simulink model "AariaHIABTorqueR2017a2"  (R2017a)
settings: Solver=VariableStepAuto  StartTime=0.0  StopTime=inf  FixedStep=0.1  RelTol=1e-3  EnableMultiTasking=on
model workspace (MATLAB code in the model file):
  | my_a =1;
undefined symbols (not defined in the file or in its folder): AARIAENV, AARIAMAN, AARIASEN, Camera, sensor, Source_TS, X, Y, Z
libraries: sm_lib x369, nesl_utility x225, dspmathops x92, simulink x70, powerlib_meascontrol x3, vrlib x2, aerolibanimutils x1, aerolibutil x1
(part 6 of 10)

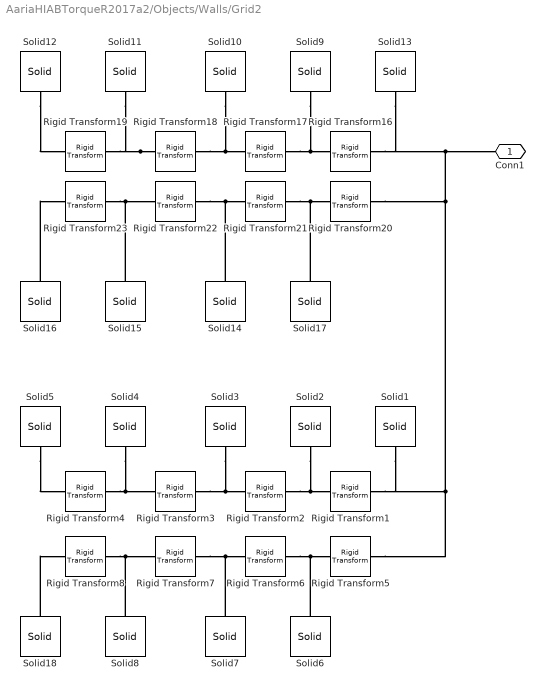
== system AariaHIABTorqueR2017a2/Objects/Walls/Grid2 ==
  Rigid Transform{1..4} (4 alike) : sm_lib/Frames and Transforms/Rigid Transform  TranslationMethod=StandardAxis  TranslationStandardOffset=2  TranslationLengthUnit=m  TranslationStandardAxis=+Y  TranslationCartesianOffset=[0 0 0]  TranslationROffset=0  TranslationROffsetUnits=m  TranslationZOffset=0  TranslationZOffsetUnits=m  TranslationThetaOffset=0  TranslationThetaOffsetUnits=deg  RotationMethod=None  RotationAngleUnits=deg  RotationStandardAxis=+Z  RotationAngle=0.0  RotationArbitraryAxis=[0 0 1]  FollAlignAxisA=+X  BaseAlignAxisA=+Y  FollAlignAxisB=+Y  BaseAlignAxisB=+Z  RotationSequenceAxes=FollowerAxes  RotationSequence=XYX  RotationSequenceAngles=[0 0 0]  RotationSequenceAnglesUnits=deg  RotationMatrix=[1 0 0; 0 1 0; 0 0 1]
  Rigid Transform{16..19} (4 alike) : sm_lib/Frames and Transforms/Rigid Transform  TranslationMethod=StandardAxis  TranslationStandardOffset=2  TranslationLengthUnit=m  TranslationStandardAxis=+X  TranslationCartesianOffset=[0 0 0]  TranslationROffset=0  TranslationROffsetUnits=m  TranslationZOffset=0  TranslationZOffsetUnits=m  TranslationThetaOffset=0  TranslationThetaOffsetUnits=deg  RotationMethod=None  RotationAngleUnits=deg  RotationStandardAxis=+Z  RotationAngle=0.0  RotationArbitraryAxis=[0 0 1]  FollAlignAxisA=+X  BaseAlignAxisA=+Y  FollAlignAxisB=+Y  BaseAlignAxisB=+Z  RotationSequenceAxes=FollowerAxes  RotationSequence=XYX  RotationSequenceAngles=[0 0 0]  RotationSequenceAnglesUnits=deg  RotationMatrix=[1 0 0; 0 1 0; 0 0 1]
  Rigid Transform{20..23} (4 alike) : sm_lib/Frames and Transforms/Rigid Transform  TranslationMethod=StandardAxis  TranslationStandardOffset=2  TranslationLengthUnit=m  TranslationStandardAxis=-X  TranslationCartesianOffset=[0 0 0]  TranslationROffset=0  TranslationROffsetUnits=m  TranslationZOffset=0  TranslationZOffsetUnits=m  TranslationThetaOffset=0  TranslationThetaOffsetUnits=deg  RotationMethod=None  RotationAngleUnits=deg  RotationStandardAxis=+Z  RotationAngle=0.0  RotationArbitraryAxis=[0 0 1]  FollAlignAxisA=+X  BaseAlignAxisA=+Y  FollAlignAxisB=+Y  BaseAlignAxisB=+Z  RotationSequenceAxes=FollowerAxes  RotationSequence=XYX  RotationSequenceAngles=[0 0 0]  RotationSequenceAnglesUnits=deg  RotationMatrix=[1 0 0; 0 1 0; 0 0 1]
  Rigid Transform{5..8} (4 alike) : sm_lib/Frames and Transforms/Rigid Transform  TranslationMethod=StandardAxis  TranslationStandardOffset=2  TranslationLengthUnit=m  TranslationStandardAxis=-Y  TranslationCartesianOffset=[0 0 0]  TranslationROffset=0  TranslationROffsetUnits=m  TranslationZOffset=0  TranslationZOffsetUnits=m  TranslationThetaOffset=0  TranslationThetaOffsetUnits=deg  RotationMethod=None  RotationAngleUnits=deg  RotationStandardAxis=+Z  RotationAngle=0.0  RotationArbitraryAxis=[0 0 1]  FollAlignAxisA=+X  BaseAlignAxisA=+Y  FollAlignAxisB=+Y  BaseAlignAxisB=+Z  RotationSequenceAxes=FollowerAxes  RotationSequence=XYX  RotationSequenceAngles=[0 0 0]  RotationSequenceAnglesUnits=deg  RotationMatrix=[1 0 0; 0 1 0; 0 0 1]
  Solid{1..8,18} (9 alike) : sm_lib/Body Elements/Solid  InertiaType=CalculateFromGeometry  Mass=1  MassUnits=kg  CenterOfMass=[0 0 0]  CenterOfMassUnits=m  MomentsOfInertia=[1 1 1]  MomentsOfInertiaUnits=kg*m^2  ProductsOfInertia=[1 1 1]  ProductsOfInertiaUnits=kg*m^2  DensityBased=on  Density=1000  DensityUnits=kg/m^3  DoExposeReferenceFrame=on  SerializedFrames=<Frames/>  GraphicType=FromGeometry  MarkerShape=Sphere  MarkerSize=10  GraphicVisPropType=SimpleVisualProperties  GraphicDiffuseColor=[0.4 0.4 0.4]  GraphicSpecularColor=[0.5 0.5 0.5 1.0]  GraphicAmbientColor=[0.15 0.15 0.15 1.0]  GraphicEmissiveColor=[0.0 0.0 0.0 1.0]  GraphicShininess=75  GraphicOpacity=1.0  GeometryShape=Brick  RectangleSize=[1 1]  RectangleSizeUnits=m  BrickDimensions=[20 1 0.12]  BrickDimensionUnits=m  CylinderRadius=1  CylinderRadiusUnits=m  CylinderLength=1  CylinderLengthUnits=m  SphereRadius=1  SphereRadiusUnits=m  EllipsoidRadii=[1 1 1]  EllipsoidRadiiUnits=m  ExtrusionCrossSection=[1 1; -1 1; -1 -1; 1 -1]  ExtrusionCrossSectionUnits=m  ExtrusionLength=1  ExtrusionLengthUnits=m  PolygonNumSides=3  PolygonOuterRadius=1  PolygonOuterRadiusUnits=m  ExtGeomFileType=STEP  ExtGeomFileUnits=m  RevolutionCrossSection=[1 1; 1 -1; 2 -1; 2 1]  RevolutionCrossSectionUnits=m  RevolutionExtent=Full  RevolutionAngle=180  RevolutionAngleUnits=deg
  Solid{9..17} (9 alike) : sm_lib/Body Elements/Solid  InertiaType=CalculateFromGeometry  Mass=1  MassUnits=kg  CenterOfMass=[0 0 0]  CenterOfMassUnits=m  MomentsOfInertia=[1 1 1]  MomentsOfInertiaUnits=kg*m^2  ProductsOfInertia=[1 1 1]  ProductsOfInertiaUnits=kg*m^2  DensityBased=on  Density=1000  DensityUnits=kg/m^3  DoExposeReferenceFrame=on  SerializedFrames=<Frames/>  GraphicType=FromGeometry  MarkerShape=Sphere  MarkerSize=10  GraphicVisPropType=SimpleVisualProperties  GraphicDiffuseColor=[0.2 0.2 0.2]  GraphicSpecularColor=[0.5 0.5 0.5 1.0]  GraphicAmbientColor=[0.15 0.15 0.15 1.0]  GraphicEmissiveColor=[0.0 0.0 0.0 1.0]  GraphicShininess=75  GraphicOpacity=1.0  GeometryShape=Brick  RectangleSize=[1 1]  RectangleSizeUnits=m  BrickDimensions=[1 20 0.11]  BrickDimensionUnits=m  CylinderRadius=1  CylinderRadiusUnits=m  CylinderLength=1  CylinderLengthUnits=m  SphereRadius=1  SphereRadiusUnits=m  EllipsoidRadii=[1 1 1]  EllipsoidRadiiUnits=m  ExtrusionCrossSection=[1 1; -1 1; -1 -1; 1 -1]  ExtrusionCrossSectionUnits=m  ExtrusionLength=1  ExtrusionLengthUnits=m  PolygonNumSides=3  PolygonOuterRadius=1  PolygonOuterRadiusUnits=m  ExtGeomFileType=STEP  ExtGeomFileUnits=m  RevolutionCrossSection=[1 1; 1 -1; 2 -1; 2 1]  RevolutionCrossSectionUnits=m  RevolutionExtent=Full  RevolutionAngle=180  RevolutionAngleUnits=deg
  Conn1 : PMIOPort  Port=1  Side=Right
  connections:
  Solid12/RConn1 -- Rigid Transform19/RConn1
  Rigid Transform18/RConn1 -- Rigid Transform19/LConn1 -- Solid11/RConn1
  Rigid Transform5/LConn1 -- Rigid Transform20/LConn1 -- Conn1/RConn1 -- Solid13/RConn1 -- Rigid Transform16/LConn1 -- Rigid Transform1/LConn1 -- Solid1/RConn1
  Rigid Transform21/LConn1 -- Rigid Transform20/RConn1 -- Solid17/RConn1
  Rigid Transform18/LConn1 -- Rigid Transform17/RConn1 -- Solid10/RConn1
  Solid15/RConn1 -- Rigid Transform23/LConn1 -- Rigid Transform22/RConn1
  Rigid Transform22/LConn1 -- Solid14/RConn1 -- Rigid Transform21/RConn1
  Rigid Transform17/LConn1 -- Rigid Transform16/RConn1 -- Solid9/RConn1
  Solid16/RConn1 -- Rigid Transform23/RConn1
  Rigid Transform2/LConn1 -- Solid2/RConn1 -- Rigid Transform1/RConn1
  Rigid Transform3/LConn1 -- Solid3/RConn1 -- Rigid Transform2/RConn1
  Solid4/RConn1 -- Rigid Transform4/LConn1 -- Rigid Transform3/RConn1
  Solid5/RConn1 -- Rigid Transform4/RConn1
  Rigid Transform6/LConn1 -- Rigid Transform5/RConn1 -- Solid6/RConn1
  Rigid Transform7/LConn1 -- Solid7/RConn1 -- Rigid Transform6/RConn1
  Rigid Transform8/LConn1 -- Solid8/RConn1 -- Rigid Transform7/RConn1
  Solid18/RConn1 -- Rigid Transform8/RConn1

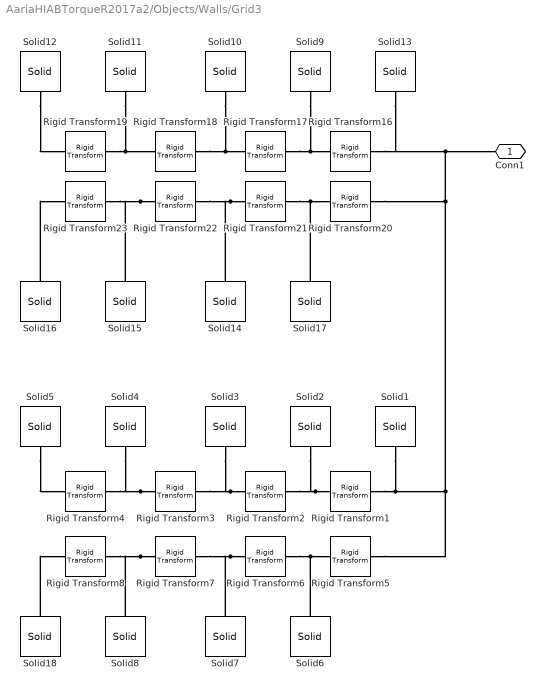
== system AariaHIABTorqueR2017a2/Objects/Walls/Grid3 ==
  Rigid Transform{1..4} (4 alike) : sm_lib/Frames and Transforms/Rigid Transform  TranslationMethod=StandardAxis  TranslationStandardOffset=2  TranslationLengthUnit=m  TranslationStandardAxis=+Y  TranslationCartesianOffset=[0 0 0]  TranslationROffset=0  TranslationROffsetUnits=m  TranslationZOffset=0  TranslationZOffsetUnits=m  TranslationThetaOffset=0  TranslationThetaOffsetUnits=deg  RotationMethod=None  RotationAngleUnits=deg  RotationStandardAxis=+Z  RotationAngle=0.0  RotationArbitraryAxis=[0 0 1]  FollAlignAxisA=+X  BaseAlignAxisA=+Y  FollAlignAxisB=+Y  BaseAlignAxisB=+Z  RotationSequenceAxes=FollowerAxes  RotationSequence=XYX  RotationSequenceAngles=[0 0 0]  RotationSequenceAnglesUnits=deg  RotationMatrix=[1 0 0; 0 1 0; 0 0 1]
  Rigid Transform{16..19} (4 alike) : sm_lib/Frames and Transforms/Rigid Transform  TranslationMethod=StandardAxis  TranslationStandardOffset=2  TranslationLengthUnit=m  TranslationStandardAxis=+X  TranslationCartesianOffset=[0 0 0]  TranslationROffset=0  TranslationROffsetUnits=m  TranslationZOffset=0  TranslationZOffsetUnits=m  TranslationThetaOffset=0  TranslationThetaOffsetUnits=deg  RotationMethod=None  RotationAngleUnits=deg  RotationStandardAxis=+Z  RotationAngle=0.0  RotationArbitraryAxis=[0 0 1]  FollAlignAxisA=+X  BaseAlignAxisA=+Y  FollAlignAxisB=+Y  BaseAlignAxisB=+Z  RotationSequenceAxes=FollowerAxes  RotationSequence=XYX  RotationSequenceAngles=[0 0 0]  RotationSequenceAnglesUnits=deg  RotationMatrix=[1 0 0; 0 1 0; 0 0 1]
  Rigid Transform{20..23} (4 alike) : sm_lib/Frames and Transforms/Rigid Transform  TranslationMethod=StandardAxis  TranslationStandardOffset=2  TranslationLengthUnit=m  TranslationStandardAxis=-X  TranslationCartesianOffset=[0 0 0]  TranslationROffset=0  TranslationROffsetUnits=m  TranslationZOffset=0  TranslationZOffsetUnits=m  TranslationThetaOffset=0  TranslationThetaOffsetUnits=deg  RotationMethod=None  RotationAngleUnits=deg  RotationStandardAxis=+Z  RotationAngle=0.0  RotationArbitraryAxis=[0 0 1]  FollAlignAxisA=+X  BaseAlignAxisA=+Y  FollAlignAxisB=+Y  BaseAlignAxisB=+Z  RotationSequenceAxes=FollowerAxes  RotationSequence=XYX  RotationSequenceAngles=[0 0 0]  RotationSequenceAnglesUnits=deg  RotationMatrix=[1 0 0; 0 1 0; 0 0 1]
  Rigid Transform{5..8} (4 alike) : sm_lib/Frames and Transforms/Rigid Transform  TranslationMethod=StandardAxis  TranslationStandardOffset=2  TranslationLengthUnit=m  TranslationStandardAxis=-Y  TranslationCartesianOffset=[0 0 0]  TranslationROffset=0  TranslationROffsetUnits=m  TranslationZOffset=0  TranslationZOffsetUnits=m  TranslationThetaOffset=0  TranslationThetaOffsetUnits=deg  RotationMethod=None  RotationAngleUnits=deg  RotationStandardAxis=+Z  RotationAngle=0.0  RotationArbitraryAxis=[0 0 1]  FollAlignAxisA=+X  BaseAlignAxisA=+Y  FollAlignAxisB=+Y  BaseAlignAxisB=+Z  RotationSequenceAxes=FollowerAxes  RotationSequence=XYX  RotationSequenceAngles=[0 0 0]  RotationSequenceAnglesUnits=deg  RotationMatrix=[1 0 0; 0 1 0; 0 0 1]
  Solid{1..8,18} (9 alike) : sm_lib/Body Elements/Solid  InertiaType=CalculateFromGeometry  Mass=1  MassUnits=kg  CenterOfMass=[0 0 0]  CenterOfMassUnits=m  MomentsOfInertia=[1 1 1]  MomentsOfInertiaUnits=kg*m^2  ProductsOfInertia=[1 1 1]  ProductsOfInertiaUnits=kg*m^2  DensityBased=on  Density=1000  DensityUnits=kg/m^3  DoExposeReferenceFrame=on  SerializedFrames=<Frames/>  GraphicType=FromGeometry  MarkerShape=Sphere  MarkerSize=10  GraphicVisPropType=SimpleVisualProperties  GraphicDiffuseColor=[0.4 0.4 0.4]  GraphicSpecularColor=[0.5 0.5 0.5 1.0]  GraphicAmbientColor=[0.15 0.15 0.15 1.0]  GraphicEmissiveColor=[0.0 0.0 0.0 1.0]  GraphicShininess=75  GraphicOpacity=1.0  GeometryShape=Brick  RectangleSize=[1 1]  RectangleSizeUnits=m  BrickDimensions=[20 1 0.12]  BrickDimensionUnits=m  CylinderRadius=1  CylinderRadiusUnits=m  CylinderLength=1  CylinderLengthUnits=m  SphereRadius=1  SphereRadiusUnits=m  EllipsoidRadii=[1 1 1]  EllipsoidRadiiUnits=m  ExtrusionCrossSection=[1 1; -1 1; -1 -1; 1 -1]  ExtrusionCrossSectionUnits=m  ExtrusionLength=1  ExtrusionLengthUnits=m  PolygonNumSides=3  PolygonOuterRadius=1  PolygonOuterRadiusUnits=m  ExtGeomFileType=STEP  ExtGeomFileUnits=m  RevolutionCrossSection=[1 1; 1 -1; 2 -1; 2 1]  RevolutionCrossSectionUnits=m  RevolutionExtent=Full  RevolutionAngle=180  RevolutionAngleUnits=deg
  Solid{9..17} (9 alike) : sm_lib/Body Elements/Solid  InertiaType=CalculateFromGeometry  Mass=1  MassUnits=kg  CenterOfMass=[0 0 0]  CenterOfMassUnits=m  MomentsOfInertia=[1 1 1]  MomentsOfInertiaUnits=kg*m^2  ProductsOfInertia=[1 1 1]  ProductsOfInertiaUnits=kg*m^2  DensityBased=on  Density=1000  DensityUnits=kg/m^3  DoExposeReferenceFrame=on  SerializedFrames=<Frames/>  GraphicType=FromGeometry  MarkerShape=Sphere  MarkerSize=10  GraphicVisPropType=SimpleVisualProperties  GraphicDiffuseColor=[0.2 0.2 0.2]  GraphicSpecularColor=[0.5 0.5 0.5 1.0]  GraphicAmbientColor=[0.15 0.15 0.15 1.0]  GraphicEmissiveColor=[0.0 0.0 0.0 1.0]  GraphicShininess=75  GraphicOpacity=1.0  GeometryShape=Brick  RectangleSize=[1 1]  RectangleSizeUnits=m  BrickDimensions=[1 20 0.11]  BrickDimensionUnits=m  CylinderRadius=1  CylinderRadiusUnits=m  CylinderLength=1  CylinderLengthUnits=m  SphereRadius=1  SphereRadiusUnits=m  EllipsoidRadii=[1 1 1]  EllipsoidRadiiUnits=m  ExtrusionCrossSection=[1 1; -1 1; -1 -1; 1 -1]  ExtrusionCrossSectionUnits=m  ExtrusionLength=1  ExtrusionLengthUnits=m  PolygonNumSides=3  PolygonOuterRadius=1  PolygonOuterRadiusUnits=m  ExtGeomFileType=STEP  ExtGeomFileUnits=m  RevolutionCrossSection=[1 1; 1 -1; 2 -1; 2 1]  RevolutionCrossSectionUnits=m  RevolutionExtent=Full  RevolutionAngle=180  RevolutionAngleUnits=deg
  Conn1 : PMIOPort  Port=1  Side=Right
  connections:
  Solid18/RConn1 -- Rigid Transform8/RConn1
  Rigid Transform7/RConn1 -- Solid8/RConn1 -- Rigid Transform8/LConn1
  Rigid Transform6/RConn1 -- Solid7/RConn1 -- Rigid Transform7/LConn1
  Solid6/RConn1 -- Rigid Transform5/RConn1 -- Rigid Transform6/LConn1
  Solid5/RConn1 -- Rigid Transform4/RConn1
  Rigid Transform3/RConn1 -- Rigid Transform4/LConn1 -- Solid4/RConn1
  Rigid Transform2/RConn1 -- Solid3/RConn1 -- Rigid Transform3/LConn1
  Rigid Transform1/RConn1 -- Solid2/RConn1 -- Rigid Transform2/LConn1
  Solid16/RConn1 -- Rigid Transform23/RConn1
  Solid9/RConn1 -- Rigid Transform16/RConn1 -- Rigid Transform17/LConn1
  Rigid Transform21/RConn1 -- Solid14/RConn1 -- Rigid Transform22/LConn1
  Rigid Transform22/RConn1 -- Rigid Transform23/LConn1 -- Solid15/RConn1
  Solid10/RConn1 -- Rigid Transform17/RConn1 -- Rigid Transform18/LConn1
  Solid17/RConn1 -- Rigid Transform20/RConn1 -- Rigid Transform21/LConn1
  Solid1/RConn1 -- Rigid Transform1/LConn1 -- Rigid Transform16/LConn1 -- Solid13/RConn1 -- Conn1/RConn1 -- Rigid Transform20/LConn1 -- Rigid Transform5/LConn1
  Solid11/RConn1 -- Rigid Transform19/LConn1 -- Rigid Transform18/RConn1
  Solid12/RConn1 -- Rigid Transform19/RConn1

== system AariaHIABTorqueR2017a2/Subsystem/grab_check_cam above angled down/Subsystem ==
  CamObj : Inport
  Constant : Constant  Value=Camera.Rotation
  Matrix Multiply : Product  Multiplication=Matrix(*)
  TipObjPose : Outport
  wires:
  CamObj/1 -> Matrix Multiply/2
  Constant/1 -> Matrix Multiply/1
  Matrix Multiply/1 -> TipObjPose/1

== system AariaHIABTorqueR2017a2/Subsystem/grab_check_cam above angled down/orientation match ==
  TipCam : Inport
  CamObj : Inport  Port=2
  "TipCamRot " : Inport  Port=3
  Abs : Abs
  Constant : Constant  Value=pi
  Constant1 : Constant  Value=Camera.AzmTol
  Constant2 : Constant  Value=Camera.DstTol
  Constant3 : Constant  Value=Camera.IncTol
  Demux{,1..3} (4 alike) : Demux  Outputs=3
  Gain1 : Gain  Gain=-1
  Invert 3x3 Matrix : aerolibutil/Invert  3x3 Matrix
  Logical Operator : Logic  Inputs=3  AllPortsSameDT=off  OutDataTypeStr=boolean
  MATLAB Function : MATLAB Function  TreatAsAtomicUnit=on
  Mux : Mux  Inputs=3
  Mux1 : Mux  Inputs=3
  Relational Operator : RelationalOperator  Operator=<=  OutDataTypeStr=boolean  RndMeth=Simplest
  Relational Operator1 : RelationalOperator  Operator=<=  OutDataTypeStr=boolean  RndMeth=Simplest
  Relational Operator2 : RelationalOperator  Operator=<=  OutDataTypeStr=boolean  RndMeth=Simplest
  Scope : Scope
  Scope2 : Scope
  Sum : Sum  Inputs=-+|
  Sum1 : Sum  Inputs=+-
  Sum2 : Sum  Inputs=++|
  Sum3 : Sum  Inputs=++|
  Terminator : Terminator
  Out1 : Outport
  wires:
  TipCam/1 -> Demux/1
  Demux/1 -> Sum/2
  Constant/1 -> Sum/1
  Sum/1 -> Sum3/2
  Demux/2 -> Mux/2
  Mux/1 -> Sum1/1
  CamObj/1 -> Demux3/1
  Sum1/1 -> Scope/1, Abs/1
  Invert 3x3 Matrix/1 -> MATLAB Function/1(u)
  "TipCamRot "/1 -> Invert 3x3 Matrix/1
  MATLAB Function/1(y) -> Demux2/1
  Demux/3 -> Gain1/1
  Gain1/1 -> Mux/3
  Demux2/2 -> Sum2/1
  Demux2/3 -> Sum3/1
  Demux3/3 -> Sum2/2
  Sum2/1 -> Mux1/3
  Demux3/2 -> Mux1/2
  Demux3/1 -> Mux1/1
  Mux1/1 -> Sum1/2
  Constant1/1 -> Relational Operator/2
  Constant2/1 -> Relational Operator1/2
  Constant3/1 -> Relational Operator2/2
  Relational Operator2/1 -> Logical Operator/3
  Relational Operator1/1 -> Logical Operator/2
  Relational Operator/1 -> Logical Operator/1
  Logical Operator/1 -> Scope2/1, Out1/1
  Demux1/1 -> Relational Operator/1
  Demux1/2 -> Relational Operator1/1
  Demux1/3 -> Relational Operator2/1
  Abs/1 -> Demux1/1
  Demux2/1 -> Terminator/1
  Sum3/1 -> Mux/1

== system AariaHIABTorqueR2017a2/Subsystem/grab_check_cam above angled down/orientation match1 ==
  TipCam : Inport
  CamObj : Inport  Port=2
  Abs : Abs
  Constant1 : Constant  Value=Camera.AzmTol
  Constant2 : Constant  Value=Camera.DstTol
  Constant3 : Constant  Value=Camera.IncTol
  Demux : Demux  Outputs=3
  Demux1 : Demux  Outputs=3
  Demux3 : Demux  Outputs=3
  Gain : Gain  Gain=-1
  Logical Operator : Logic  Inputs=3  AllPortsSameDT=off  OutDataTypeStr=boolean
  Mux : Mux  Inputs=3
  Mux1 : Mux  Inputs=3
  Relational Operator : RelationalOperator  Operator=<=  OutDataTypeStr=boolean  RndMeth=Simplest
  Relational Operator1 : RelationalOperator  Operator=<=  OutDataTypeStr=boolean  RndMeth=Simplest
  Relational Operator2 : RelationalOperator  Operator=<=  OutDataTypeStr=boolean  RndMeth=Simplest
  Sum : Sum  Inputs=+++
  Sum1 : Sum  Inputs=+-
  Out1 : Outport
  Orient_penalty : Outport  Port=2
  wires:
  Demux/1 -> Mux/1
  Abs/1 -> Demux1/1
  Demux1/3 -> Sum/3, Relational Operator2/1
  Demux1/2 -> Sum/2, Relational Operator1/1
  Demux1/1 -> Sum/1, Relational Operator/1
  Logical Operator/1 -> Out1/1
  Relational Operator/1 -> Logical Operator/1
  Relational Operator1/1 -> Logical Operator/2
  Relational Operator2/1 -> Logical Operator/3
  Constant3/1 -> Relational Operator2/2
  Constant2/1 -> Relational Operator1/2
  Constant1/1 -> Relational Operator/2
  Mux1/1 -> Sum1/2
  Demux3/1 -> Mux1/1
  Demux3/2 -> Mux1/2
  Demux3/3 -> Mux1/3
  Demux/3 -> Mux/3
  Sum1/1 -> Abs/1
  CamObj/1 -> Demux3/1
  Mux/1 -> Sum1/1
  Demux/2 -> Mux/2
  TipCam/1 -> Demux/1
  Sum/1 -> Gain/1
  Gain/1 -> Orient_penalty/1

== system AariaHIABTorqueR2017a2/Subsystem/grab_check_cam above angled down/pose match ==
  Obj_pose : Inport
  Abs : Abs
  Abs1 : Abs
  Abs2 : Abs
  Constant3 : Constant
  Constant4 : Constant  Value=[1:3]
  Constant5 : Constant  Value=2
  Constant6 : Constant  Value=[1:3]
  Constant7 : Constant  Value=3
  Constant8 : Constant  Value=[1:3]
  Constant9 : Constant  Value=Camera.PickRotation
  Logical Operator : Logic  Inputs=3  AllPortsSameDT=off  OutDataTypeStr=boolean
  Max : MinMax  Function=max
  Max1 : MinMax  Function=max
  Max2 : MinMax  Function=max
  Relational Operator : RelationalOperator  OutDataTypeStr=boolean  RndMeth=Simplest
  Relational Operator1 : RelationalOperator  OutDataTypeStr=boolean  RndMeth=Simplest
  Relational Operator2 : RelationalOperator  OutDataTypeStr=boolean  RndMeth=Simplest
  Scope : Scope
  Selector : Selector  NumberOfDimensions=2  InputPortWidth=3  IndexOptions=Index vector (port),Index vector (port)  Indices=1,1  OutputSizes=1,1
  Selector1 : Selector  NumberOfDimensions=2  InputPortWidth=3  IndexOptions=Index vector (port),Index vector (port)  Indices=1,1  OutputSizes=1,1
  Selector2 : Selector  NumberOfDimensions=2  InputPortWidth=3  IndexOptions=Index vector (port),Index vector (port)  Indices=1,1  OutputSizes=1,1
  Sum : Sum  Inputs=+++
  grab_pose_ok : Outport
  PoseBonus : Outport  Port=2
  wires:
  Constant4/1 -> Selector/3
  Constant7/1 -> Selector2/2
  Selector2/1 -> Abs2/1
  Constant8/1 -> Selector2/3
  Constant9/1 -> Relational Operator/2, Relational Operator1/2, Relational Operator2/2
  Constant3/1 -> Selector/2
  Relational Operator/1 -> Logical Operator/1
  Relational Operator1/1 -> Logical Operator/2
  Logical Operator/1 -> Scope/1, grab_pose_ok/1
  Selector1/1 -> Abs1/1
  Max/1 -> Sum/1, Relational Operator/1
  Abs1/1 -> Max1/1
  Abs2/1 -> Max2/1
  Max1/1 -> Sum/2, Relational Operator1/1
  Relational Operator2/1 -> Logical Operator/3
  Selector/1 -> Abs/1
  Max2/1 -> Sum/3, Relational Operator2/1
  Constant6/1 -> Selector1/3
  Constant5/1 -> Selector1/2
  Obj_pose/1 -> Selector/1, Selector1/1, Selector2/1
  Abs/1 -> Max/1
  Sum/1 -> PoseBonus/1

== system AariaHIABTorqueR2017a2/Tool/IMU Tool/Sensor Module1 ==
  Gain : Gain  Gain=1/AARIAENV.Min_TS
  Gain1 : Gain  Gain=1/AARIAENV.Min_TS^2
  Gain3 : Gain  Gain=AARIAENV.gravity  Multiplication=Matrix(K*u)
  Mux : Mux  Inputs=3
  Mux1 : Mux  Inputs=3
  Mux2 : Mux  Inputs=3
  PS-Simulink Converter{5..11} (7 alike) : nesl_utility/PS-Simulink Converter  PhysicalDomain=network_engine_domain  SubClassName=ps_output  LeftPortType=input  RightPortType=output  PseudoPeriodic=off  Frequencies=[]  Unit=1  AffineConversion=off
  PS-Simulink Converter2 : nesl_utility/PS-Simulink Converter  PhysicalDomain=network_engine_domain  SubClassName=ps_output  LeftPortType=input  RightPortType=output  PseudoPeriodic=off  Frequencies=[]  Unit=rad/s  AffineConversion=off
  PS-Simulink Converter3 : nesl_utility/PS-Simulink Converter  PhysicalDomain=network_engine_domain  SubClassName=ps_output  LeftPortType=input  RightPortType=output  PseudoPeriodic=off  Frequencies=[]  Unit=rad/s  AffineConversion=off
  PS-Simulink Converter4 : nesl_utility/PS-Simulink Converter  PhysicalDomain=network_engine_domain  SubClassName=ps_output  LeftPortType=input  RightPortType=output  PseudoPeriodic=off  Frequencies=[]  Unit=rad/s  AffineConversion=off
  Sensor Place : sm_lib/Frames and Transforms/Rigid Transform  TranslationMethod=Cartesian  TranslationStandardOffset=0  TranslationLengthUnit=m  TranslationStandardAxis=+Z  TranslationCartesianOffset=AARIAMAN.L(nL).S(nS).pose_p  TranslationROffset=0  TranslationROffsetUnits=m  TranslationZOffset=0  TranslationZOffsetUnits=m  TranslationThetaOffset=0  TranslationThetaOffsetUnits=deg  RotationMethod=RotationMatrix  RotationAngleUnits=deg  RotationStandardAxis=+Z  RotationAngle=0.0  RotationArbitraryAxis=[0 0 1]  FollAlignAxisA=+X  BaseAlignAxisA=+Y  FollAlignAxisB=+Y  BaseAlignAxisB=+Z  RotationSequenceAxes=FollowerAxes  RotationSequence=XYX  RotationSequenceAngles=[0 0 0]  RotationSequenceAnglesUnits=deg  RotationMatrix=AARIAMAN.L(nL).S(nS).pose_r
  Sum : Sum  Inputs=|++
  Sum1 : Sum  Inputs=|++
  Sum2 : Sum  Inputs=++|
  Transform Sensor : sm_lib/Frames and Transforms/Transform Sensor  MeasurementFrame=Follower  SenseAngle=off  SenseAxis=off  SenseAngle1=off  SenseAngle2=off  SenseAngle3=off  SenseQ=off  SenseR=on  SenseOmegaX=on  SenseOmegaY=on  SenseOmegaZ=on  SenseOmega1=off  SenseOmega2=off  SenseOmega3=off  SenseQDot=off  SenseRDot=off  SenseAlphaX=off  SenseAlphaY=off  SenseAlphaZ=off  SenseAlpha1=off  SenseAlpha2=off  SenseAlpha3=off  SenseQDDot=off  SenseRDDot=off  SenseX=on  SenseY=on  SenseZ=on  SenseRad=off  SenseAzim=off  SenseDist=off  SenseInc=off  SenseXDot=off  SenseYDot=off  SenseZDot=off  SenseRadDot=off  SenseAzimDot=off  SenseDistDot=off  SenseIncDot=off  SenseXDDot=on  SenseYDDot=on  SenseZDDot=on  SenseRadDDot=off  SenseAzimDDot=off  SenseDistDDot=off  SenseIncDDot=off
  a_noise : Subsystem
  coord_sens : sm_lib/Body Elements/Graphic  GraphicType=Marker  MarkerShape=Frame  MarkerSize=AARIAMAN.vis.coord_sizeS  GraphicVisPropType=SimpleVisualProperties  GraphicDiffuseColor=AARIAMAN.vis.col_s  GraphicSpecularColor=[0.5 0.5 0.5 1.0]  GraphicAmbientColor=[0.15 0.15 0.15 1.0]  GraphicEmissiveColor=[0.0 0.0 0.0 1.0]  GraphicShininess=75  GraphicOpacity=AARIAMAN.vis.opacity_s
      settings: SourceProductName=Simscape Multibody
  omega_noise : Subsystem
  Body Frame : PMIOPort  Port=1  Side=Left
  Reference Frame : PMIOPort  Port=2  Side=Left
  Out5 : Outport
  Out4 : Outport  Port=2
  Out2 : Outport  Port=3
  Out3 : Outport  Port=4
  wires:
  Sum2/1 -> Out5/1  "omega_measured"
  Sum/1 -> Sum1/1
  PS-Simulink Converter8/1 -> Gain3/1, Out3/1  "R_actual"
  Mux2/1 -> Gain1/1
  PS-Simulink Converter7/1 -> Mux1/3
  PS-Simulink Converter5/1 -> Mux1/1
  PS-Simulink Converter6/1 -> Mux1/2
  Mux/1 -> Gain/1
  PS-Simulink Converter4/1 -> Mux/3
  PS-Simulink Converter2/1 -> Mux/1
  PS-Simulink Converter3/1 -> Mux/2
  PS-Simulink Converter9/1 -> Mux2/1
  PS-Simulink Converter11/1 -> Mux2/3
  Mux1/1 -> Out2/1  "P_actual"
  PS-Simulink Converter10/1 -> Mux2/2
  Sum1/1 -> Out4/1  "a_measured"
  Gain3/1 -> Sum/2  "a_measured"
  omega_noise/1(noise) -> Sum2/1
  a_noise/1(noise) -> Sum1/2
  Gain/1 -> Sum2/2
  Gain1/1 -> Sum/1
  connections:
  Transform Sensor/RConn7 -- PS-Simulink Converter6/LConn1
  Transform Sensor/RConn8 -- PS-Simulink Converter7/LConn1
  PS-Simulink Converter8/LConn1 -- Transform Sensor/RConn2
  Transform Sensor/RConn6 -- PS-Simulink Converter5/LConn1
  Transform Sensor/RConn10 -- PS-Simulink Converter10/LConn1
  Transform Sensor/RConn5 -- PS-Simulink Converter4/LConn1
  Transform Sensor/LConn1 -- Reference Frame/RConn1
  Transform Sensor/RConn4 -- PS-Simulink Converter3/LConn1
  Transform Sensor/RConn9 -- PS-Simulink Converter9/LConn1
  Transform Sensor/RConn3 -- PS-Simulink Converter2/LConn1
  Sensor Place/LConn1 -- Body Frame/RConn1
  Transform Sensor/RConn11 -- PS-Simulink Converter11/LConn1
  Transform Sensor/RConn1 -- coord_sens/RConn1 -- Sensor Place/RConn1

== system AariaHIABTorqueR2017a2/Tool/IMU Tool1/Sensor Module1 ==
  Gain : Gain  Gain=1/AARIAENV.Min_TS
  Gain1 : Gain  Gain=1/AARIAENV.Min_TS^2
  Gain3 : Gain  Gain=AARIAENV.gravity  Multiplication=Matrix(K*u)
  Mux : Mux  Inputs=3
  Mux1 : Mux  Inputs=3
  Mux2 : Mux  Inputs=3
  PS-Simulink Converter{5..11} (7 alike) : nesl_utility/PS-Simulink Converter  PhysicalDomain=network_engine_domain  SubClassName=ps_output  LeftPortType=input  RightPortType=output  PseudoPeriodic=off  Frequencies=[]  Unit=1  AffineConversion=off
  PS-Simulink Converter2 : nesl_utility/PS-Simulink Converter  PhysicalDomain=network_engine_domain  SubClassName=ps_output  LeftPortType=input  RightPortType=output  PseudoPeriodic=off  Frequencies=[]  Unit=rad/s  AffineConversion=off
  PS-Simulink Converter3 : nesl_utility/PS-Simulink Converter  PhysicalDomain=network_engine_domain  SubClassName=ps_output  LeftPortType=input  RightPortType=output  PseudoPeriodic=off  Frequencies=[]  Unit=rad/s  AffineConversion=off
  PS-Simulink Converter4 : nesl_utility/PS-Simulink Converter  PhysicalDomain=network_engine_domain  SubClassName=ps_output  LeftPortType=input  RightPortType=output  PseudoPeriodic=off  Frequencies=[]  Unit=rad/s  AffineConversion=off
  Sensor Place : sm_lib/Frames and Transforms/Rigid Transform  TranslationMethod=Cartesian  TranslationStandardOffset=0  TranslationLengthUnit=m  TranslationStandardAxis=+Z  TranslationCartesianOffset=AARIAMAN.L(nL).S(nS).pose_p  TranslationROffset=0  TranslationROffsetUnits=m  TranslationZOffset=0  TranslationZOffsetUnits=m  TranslationThetaOffset=0  TranslationThetaOffsetUnits=deg  RotationMethod=RotationMatrix  RotationAngleUnits=deg  RotationStandardAxis=+Z  RotationAngle=0.0  RotationArbitraryAxis=[0 0 1]  FollAlignAxisA=+X  BaseAlignAxisA=+Y  FollAlignAxisB=+Y  BaseAlignAxisB=+Z  RotationSequenceAxes=FollowerAxes  RotationSequence=XYX  RotationSequenceAngles=[0 0 0]  RotationSequenceAnglesUnits=deg  RotationMatrix=AARIAMAN.L(nL).S(nS).pose_r
  Sum : Sum  Inputs=|++
  Sum1 : Sum  Inputs=|++
  Sum2 : Sum  Inputs=++|
  Transform Sensor : sm_lib/Frames and Transforms/Transform Sensor  MeasurementFrame=World  SenseAngle=off  SenseAxis=off  SenseAngle1=off  SenseAngle2=off  SenseAngle3=off  SenseQ=off  SenseR=on  SenseOmegaX=on  SenseOmegaY=on  SenseOmegaZ=on  SenseOmega1=off  SenseOmega2=off  SenseOmega3=off  SenseQDot=off  SenseRDot=off  SenseAlphaX=off  SenseAlphaY=off  SenseAlphaZ=off  SenseAlpha1=off  SenseAlpha2=off  SenseAlpha3=off  SenseQDDot=off  SenseRDDot=off  SenseX=on  SenseY=on  SenseZ=on  SenseRad=off  SenseAzim=off  SenseDist=off  SenseInc=off  SenseXDot=off  SenseYDot=off  SenseZDot=off  SenseRadDot=off  SenseAzimDot=off  SenseDistDot=off  SenseIncDot=off  SenseXDDot=on  SenseYDDot=on  SenseZDDot=on  SenseRadDDot=off  SenseAzimDDot=off  SenseDistDDot=off  SenseIncDDot=off
  a_noise : Subsystem
  coord_sens : sm_lib/Body Elements/Graphic  GraphicType=Marker  MarkerShape=Frame  MarkerSize=AARIAMAN.vis.coord_sizeS  GraphicVisPropType=SimpleVisualProperties  GraphicDiffuseColor=AARIAMAN.vis.col_s  GraphicSpecularColor=[0.5 0.5 0.5 1.0]  GraphicAmbientColor=[0.15 0.15 0.15 1.0]  GraphicEmissiveColor=[0.0 0.0 0.0 1.0]  GraphicShininess=75  GraphicOpacity=AARIAMAN.vis.opacity_s
      settings: SourceProductName=Simscape Multibody
  omega_noise : Subsystem
  Body Frame : PMIOPort  Port=1  Side=Left
  Reference Frame : PMIOPort  Port=2  Side=Left
  Out5 : Outport
  Out4 : Outport  Port=2
  Out2 : Outport  Port=3
  Out3 : Outport  Port=4
  wires:
  Gain1/1 -> Sum/1
  Gain/1 -> Sum2/2
  a_noise/1(noise) -> Sum1/2
  omega_noise/1(noise) -> Sum2/1
  Gain3/1 -> Sum/2  "a_measured"
  Sum1/1 -> Out4/1  "a_measured"
  PS-Simulink Converter10/1 -> Mux2/2
  Mux1/1 -> Out2/1  "P_actual"
  PS-Simulink Converter11/1 -> Mux2/3
  PS-Simulink Converter9/1 -> Mux2/1
  PS-Simulink Converter3/1 -> Mux/2
  PS-Simulink Converter2/1 -> Mux/1
  PS-Simulink Converter4/1 -> Mux/3
  Mux/1 -> Gain/1
  PS-Simulink Converter6/1 -> Mux1/2
  PS-Simulink Converter5/1 -> Mux1/1
  PS-Simulink Converter7/1 -> Mux1/3
  Mux2/1 -> Gain1/1
  PS-Simulink Converter8/1 -> Out3/1, Gain3/1  "R_actual"
  Sum/1 -> Sum1/1
  Sum2/1 -> Out5/1  "omega_measured"
  connections:
  Sensor Place/RConn1 -- coord_sens/RConn1 -- Transform Sensor/RConn1
  Transform Sensor/RConn11 -- PS-Simulink Converter11/LConn1
  Sensor Place/LConn1 -- Body Frame/RConn1
  Transform Sensor/RConn3 -- PS-Simulink Converter2/LConn1
  Transform Sensor/RConn9 -- PS-Simulink Converter9/LConn1
  Transform Sensor/RConn4 -- PS-Simulink Converter3/LConn1
  Transform Sensor/LConn1 -- Reference Frame/RConn1
  Transform Sensor/RConn5 -- PS-Simulink Converter4/LConn1
  Transform Sensor/RConn10 -- PS-Simulink Converter10/LConn1
  Transform Sensor/RConn6 -- PS-Simulink Converter5/LConn1
  PS-Simulink Converter8/LConn1 -- Transform Sensor/RConn2
  Transform Sensor/RConn8 -- PS-Simulink Converter7/LConn1
  Transform Sensor/RConn7 -- PS-Simulink Converter6/LConn1

== system AariaHIABTorqueR2017a2/Tool Sensors/Camera sensor/omega_noise ==
  Constant3 : Constant  Value=sensor.gMu
  Constant4 : Constant  Value=sensor.gSigma
  Cumulative Sum : dspmathops/Cumulative Sum  dim=Channels (running sum)  InputProcessing=Columns as channels (frame based)  reset_popup=None  outputDataTypeStr=Inherit: Same as accumulator  outputLastDataTypeStr=Inherit: Same as accumulator  outputMin=[]  outputMax=[]  roundingMode=Floor  overflowMode=off
      settings: SourceProductName=DSP System Toolbox
  Gain1 : Gain  Gain=sensor.ErrorGain
  Mux5 : Mux  Inputs=3
  Normally_distributed_random : MATLAB Function  TreatAsAtomicUnit=on
  Sum3 : Sum  Inputs=+++
  gyro in-run bias : simulink/Sources/Ramp  slope=sensor.gBias  start=0  X0=sensor.gInitBias
  gyro random walk : UniformRandomNumber  Minimum=-sensor.gWalk  Maximum=sensor.gWalk  Seed=sensor.gWalkSeed  SampleTime=Source_TS
  noise : Outport
  wires:
  gyro random walk/1 -> Cumulative Sum/1
  Normally_distributed_random/1(y) -> Sum3/2
  Cumulative Sum/1 -> Sum3/3
  Mux5/1 -> noise/1
  Constant4/1 -> Normally_distributed_random/2(sigma)
  Gain1/1 -> Mux5/3, Mux5/1, Mux5/2
  gyro in-run bias/1 -> Sum3/1
  Sum3/1 -> Gain1/1
  Constant3/1 -> Normally_distributed_random/1(mu)

== system AariaHIABTorqueR2017a2/Tool Sensors/Camera sensor/placeholder noise 3 ==
  Mux : Mux  Inputs=3
  Uniform Random Number : UniformRandomNumber  Minimum=-0.01  Maximum=0.01  SampleTime=0.1
  noise : Outport
  wires:
  Mux/1 -> noise/1
  Uniform Random Number/1 -> Mux/3, Mux/1, Mux/2

== system AariaHIABTorqueR2017a2/Tool Sensors/Camera sensor/placeholder noise1 ==
  Mux : Mux  Inputs=3
  Uniform Random Number : UniformRandomNumber  Minimum=-0.01  Maximum=0.01  SampleTime=0.1
  noise : Outport
  wires:
  Uniform Random Number/1 -> Mux/2, Mux/1, Mux/3
  Mux/1 -> noise/1

== system AariaHIABTorqueR2017a2/Tool Sensors/Camera sensor/placeholder noise2 ==
  Constant : Constant  Value=[1 1 1; 1 1 1; 1 1 1]
  Product : Product
  Uniform Random Number : UniformRandomNumber  Minimum=-0.01  Maximum=0.01  SampleTime=0.1
  noise : Outport
  wires:
  Uniform Random Number/1 -> Product/2
  Product/1 -> noise/1
  Constant/1 -> Product/1

== system AariaHIABTorqueR2017a2/Tool Sensors/Object tracker/Subsystem ==
  Camera rotation : Inport
  Object rotation : Inport  Port=2
  Matrix Multiply : Product  Multiplication=Matrix(*)
  Object world pose : Outport
  wires:
  Object rotation/1 -> Matrix Multiply/2
  Camera rotation/1 -> Matrix Multiply/1
  Matrix Multiply/1 -> Object world pose/1

== system AariaHIABTorqueR2017a2/Tool Sensors/Object tracker/placeholder noise1 ==
  Uniform Random Number : UniformRandomNumber  Minimum=-0.1  Maximum=0.1  Seed=1  SampleTime=0.1
  noise : Outport
  wires:
  Uniform Random Number/1 -> noise/1

== system AariaHIABTorqueR2017a2/Tool Sensors/Object tracker/placeholder noise2 ==
  Uniform Random Number : UniformRandomNumber  Minimum=-0.1  Maximum=0.1  Seed=2  SampleTime=0.1
  noise : Outport
  wires:
  Uniform Random Number/1 -> noise/1

== system AariaHIABTorqueR2017a2/Tool Sensors/Object tracker/placeholder noise3 ==
  Uniform Random Number : UniformRandomNumber  Minimum=-0.1  Maximum=0.1  SampleTime=0.1
  noise : Outport
  wires:
  Uniform Random Number/1 -> noise/1

== system AariaHIABTorqueR2017a2/Tool Sensors/Tool sensor1/omega_noise ==
  Constant3 : Constant  Value=sensor.gMu
  Constant4 : Constant  Value=sensor.gSigma
  Cumulative Sum : dspmathops/Cumulative Sum  dim=Channels (running sum)  InputProcessing=Columns as channels (frame based)  reset_popup=None  outputDataTypeStr=Inherit: Same as accumulator  outputLastDataTypeStr=Inherit: Same as accumulator  outputMin=[]  outputMax=[]  roundingMode=Floor  overflowMode=off
      settings: SourceProductName=DSP System Toolbox
  Gain1 : Gain  Gain=sensor.ErrorGain
  Mux5 : Mux  Inputs=3
  Normally_distributed_random : MATLAB Function  TreatAsAtomicUnit=on
  Sum3 : Sum  Inputs=+++
  gyro in-run bias : simulink/Sources/Ramp  slope=sensor.gBias  start=0  X0=sensor.gInitBias
  gyro random walk : UniformRandomNumber  Minimum=-sensor.gWalk  Maximum=sensor.gWalk  Seed=sensor.gWalkSeed  SampleTime=Source_TS
  noise : Outport
  wires:
  gyro random walk/1 -> Cumulative Sum/1
  Normally_distributed_random/1(y) -> Sum3/2
  Cumulative Sum/1 -> Sum3/3
  Mux5/1 -> noise/1
  Constant4/1 -> Normally_distributed_random/2(sigma)
  Gain1/1 -> Mux5/3, Mux5/1, Mux5/2
  gyro in-run bias/1 -> Sum3/1
  Sum3/1 -> Gain1/1
  Constant3/1 -> Normally_distributed_random/1(mu)

== system AariaHIABTorqueR2017a2/Tool Sensors/Tool sensor1/placeholder noise 3 ==
  Mux : Mux  Inputs=3
  Uniform Random Number : UniformRandomNumber  Minimum=-0.01  Maximum=0.01  SampleTime=0.1
  noise : Outport
  wires:
  Mux/1 -> noise/1
  Uniform Random Number/1 -> Mux/3, Mux/1, Mux/2

== system AariaHIABTorqueR2017a2/Tool Sensors/Tool sensor1/placeholder noise1 ==
  Mux : Mux  Inputs=3
  Uniform Random Number : UniformRandomNumber  Minimum=-0.01  Maximum=0.01  SampleTime=0.1
  noise : Outport
  wires:
  Uniform Random Number/1 -> Mux/2, Mux/1, Mux/3
  Mux/1 -> noise/1

== system AariaHIABTorqueR2017a2/Tool Sensors/Tool sensor1/placeholder noise2 ==
  Constant : Constant  Value=[1 1 1; 1 1 1; 1 1 1]
  Product : Product
  Uniform Random Number : UniformRandomNumber  Minimum=-0.01  Maximum=0.01  SampleTime=0.1
  noise : Outport
  wires:
  Uniform Random Number/1 -> Product/2
  Product/1 -> noise/1
  Constant/1 -> Product/1

== system AariaHIABTorqueR2017a2/Tool Sensors/Tool sensor2/placeholder noise 3 ==
  Mux : Mux  Inputs=3
  Uniform Random Number : UniformRandomNumber  Minimum=-0.01  Maximum=0.01  SampleTime=0.1
  noise : Outport
  wires:
  Uniform Random Number/1 -> Mux/2, Mux/1, Mux/3
  Mux/1 -> noise/1

== system AariaHIABTorqueR2017a2/Tool Sensors/Tool sensor2/placeholder noise1 ==
  Mux : Mux  Inputs=3
  Uniform Random Number : UniformRandomNumber  Minimum=-0.01  Maximum=0.01  SampleTime=0.1
  noise : Outport
  wires:
  Mux/1 -> noise/1
  Uniform Random Number/1 -> Mux/3, Mux/1, Mux/2

== system AariaHIABTorqueR2017a2/Tool Sensors/Tool sensor2/placeholder noise2 ==
  Constant : Constant  Value=[1 1 1; 1 1 1; 1 1 1]
  Product : Product
  Uniform Random Number : UniformRandomNumber  Minimum=-0.01  Maximum=0.01  SampleTime=0.1
  noise : Outport
  wires:
  Constant/1 -> Product/1
  Product/1 -> noise/1
  Uniform Random Number/1 -> Product/2

== system AariaHIABTorqueR2017a2/Base/BaseVSS/BaseEmpty/IMU Base ==
  Sensor Module1 : Subsystem  mask{nL=nL, nS=1}
      mask prompts: nL "Link Number"; nS "Sensor ID of that link"
      mask DialogControl DescGroupVar Prompt: Virtual IMU
      mask DialogControl DescTextVar Prompt: Measures Connected Body's acceleration and angular velocity in the given point
      mask DialogControl Control2 Prompt: The following numbers defines the corresponding numbers for this sensor to read from the parameters file
  Body Coord : PMIOPort  Port=1  Side=Left
  Reference Coord : PMIOPort  Port=2  Side=Left
  Out1 : Outport
  Out2 : Outport  Port=2
  Out3 : Outport  Port=3
  Out4 : Outport  Port=4
  wires:
  Sensor Module1/3(Out2) -> Out3/1
  Sensor Module1/2(Out4) -> Out2/1
  Sensor Module1/4(Out3) -> Out4/1
  Sensor Module1/1(Out5) -> Out1/1
  connections:
  Sensor Module1/LConn2 -- Reference Coord/RConn1
  Sensor Module1/LConn1 -- Body Coord/RConn1

== system AariaHIABTorqueR2017a2/Base/BaseVSS/BaseMotion/IMU Base ==
  Sensor Module1 : Subsystem  mask{nL=nL, nS=1}
      mask prompts: nL "Link Number"; nS "Sensor ID of that link"
      mask DialogControl DescGroupVar Prompt: Virtual IMU
      mask DialogControl DescTextVar Prompt: Measures Connected Body's acceleration and angular velocity in the given point
      mask DialogControl Control2 Prompt: The following numbers defines the corresponding numbers for this sensor to read from the parameters file
  Body Coord : PMIOPort  Port=1  Side=Left
  Reference Coord : PMIOPort  Port=2  Side=Left
  Out1 : Outport
  Out2 : Outport  Port=2
  Out3 : Outport  Port=3
  Out4 : Outport  Port=4
  wires:
  Sensor Module1/3(Out2) -> Out3/1
  Sensor Module1/2(Out4) -> Out2/1
  Sensor Module1/4(Out3) -> Out4/1
  Sensor Module1/1(Out5) -> Out1/1
  connections:
  Sensor Module1/LConn2 -- Reference Coord/RConn1
  Sensor Module1/LConn1 -- Body Coord/RConn1

== system AariaHIABTorqueR2017a2/Base/BaseVSS/BaseMotion/x 2motion2 ==
  X : Inport
  Difference : simulink/Discrete/Difference  ICPrevInput=1  InputProcessing=Inherited  OutMin=[]  OutMax=[]  OutDataType=fixdt(1, 16)  OutScaling=2^-10  DoSatur=off
  Difference1 : simulink/Discrete/Difference  ICPrevInput=0  InputProcessing=Inherited  OutMin=[]  OutMax=[]  OutDataType=fixdt(1, 16)  OutScaling=2^-10  DoSatur=off
  Simulink-PS Converter : nesl_utility/Simulink-PS Converter  PhysicalDomain=network_engine_domain  SubClassName=ps_input  LeftPortType=input  RightPortType=output  PseudoPeriodic=off  Frequencies=[]  NoiseDistribution=none  NoiseParameters=[]  Unit=1  AffineConversion=off  FilteringAndDerivatives=provide  SimscapeFilterOrder=1  InputFilterTimeConstant=0.001  UdotUserProvided=2
  Motion for PS : PMIOPort  Port=1  Side=Right
  wires:
  X/1 -> Simulink-PS Converter/1, Difference1/1
  Difference/1 -> Simulink-PS Converter/3
  Difference1/1 -> Difference/1, Simulink-PS Converter/2
  connections:
  Simulink-PS Converter/RConn1 -- Motion for PS/RConn1

== system AariaHIABTorqueR2017a2/Base/BaseVSS/BaseMotion/x 2motion3 ==
  X : Inport
  Difference : simulink/Discrete/Difference  ICPrevInput=1  InputProcessing=Inherited  OutMin=[]  OutMax=[]  OutDataType=fixdt(1, 16)  OutScaling=2^-10  DoSatur=off
  Difference1 : simulink/Discrete/Difference  ICPrevInput=0  InputProcessing=Inherited  OutMin=[]  OutMax=[]  OutDataType=fixdt(1, 16)  OutScaling=2^-10  DoSatur=off
  Simulink-PS Converter : nesl_utility/Simulink-PS Converter  PhysicalDomain=network_engine_domain  SubClassName=ps_input  LeftPortType=input  RightPortType=output  PseudoPeriodic=off  Frequencies=[]  NoiseDistribution=none  NoiseParameters=[]  Unit=1  AffineConversion=off  FilteringAndDerivatives=provide  SimscapeFilterOrder=1  InputFilterTimeConstant=0.001  UdotUserProvided=2
  Motion for PS : PMIOPort  Port=1  Side=Right
  wires:
  Difference1/1 -> Simulink-PS Converter/2, Difference/1
  Difference/1 -> Simulink-PS Converter/3
  X/1 -> Difference1/1, Simulink-PS Converter/1
  connections:
  Simulink-PS Converter/RConn1 -- Motion for PS/RConn1

== system AariaHIABTorqueR2017a2/Base/BaseVSS/BaseMotion/x 2motion4 ==
  X : Inport
  Difference : simulink/Discrete/Difference  ICPrevInput=1  InputProcessing=Inherited  OutMin=[]  OutMax=[]  OutDataType=fixdt(1, 16)  OutScaling=2^-10  DoSatur=off
  Difference1 : simulink/Discrete/Difference  ICPrevInput=0  InputProcessing=Inherited  OutMin=[]  OutMax=[]  OutDataType=fixdt(1, 16)  OutScaling=2^-10  DoSatur=off
  Simulink-PS Converter : nesl_utility/Simulink-PS Converter  PhysicalDomain=network_engine_domain  SubClassName=ps_input  LeftPortType=input  RightPortType=output  PseudoPeriodic=off  Frequencies=[]  NoiseDistribution=none  NoiseParameters=[]  Unit=1  AffineConversion=off  FilteringAndDerivatives=provide  SimscapeFilterOrder=1  InputFilterTimeConstant=0.001  UdotUserProvided=2
  Motion for PS : PMIOPort  Port=1  Side=Right
  wires:
  X/1 -> Simulink-PS Converter/1, Difference1/1
  Difference/1 -> Simulink-PS Converter/3
  Difference1/1 -> Difference/1, Simulink-PS Converter/2
  connections:
  Simulink-PS Converter/RConn1 -- Motion for PS/RConn1

== system AariaHIABTorqueR2017a2/Base/BaseVSS/BaseMotion/x 2motion5 ==
  X : Inport
  Difference : simulink/Discrete/Difference  ICPrevInput=1  InputProcessing=Inherited  OutMin=[]  OutMax=[]  OutDataType=fixdt(1, 16)  OutScaling=2^-10  DoSatur=off
  Difference1 : simulink/Discrete/Difference  ICPrevInput=0  InputProcessing=Inherited  OutMin=[]  OutMax=[]  OutDataType=fixdt(1, 16)  OutScaling=2^-10  DoSatur=off
  Simulink-PS Converter : nesl_utility/Simulink-PS Converter  PhysicalDomain=network_engine_domain  SubClassName=ps_input  LeftPortType=input  RightPortType=output  PseudoPeriodic=off  Frequencies=[]  NoiseDistribution=none  NoiseParameters=[]  Unit=1  AffineConversion=off  FilteringAndDerivatives=provide  SimscapeFilterOrder=1  InputFilterTimeConstant=0.001  UdotUserProvided=2
  Motion for PS : PMIOPort  Port=1  Side=Right
  wires:
  Difference1/1 -> Simulink-PS Converter/2, Difference/1
  Difference/1 -> Simulink-PS Converter/3
  X/1 -> Difference1/1, Simulink-PS Converter/1
  connections:
  Simulink-PS Converter/RConn1 -- Motion for PS/RConn1

== system AariaHIABTorqueR2017a2/Base/BaseVSS/BaseMotion/x 2motion6 ==
  X : Inport
  Difference : simulink/Discrete/Difference  ICPrevInput=1  InputProcessing=Inherited  OutMin=[]  OutMax=[]  OutDataType=fixdt(1, 16)  OutScaling=2^-10  DoSatur=off
  Difference1 : simulink/Discrete/Difference  ICPrevInput=0  InputProcessing=Inherited  OutMin=[]  OutMax=[]  OutDataType=fixdt(1, 16)  OutScaling=2^-10  DoSatur=off
  Simulink-PS Converter : nesl_utility/Simulink-PS Converter  PhysicalDomain=network_engine_domain  SubClassName=ps_input  LeftPortType=input  RightPortType=output  PseudoPeriodic=off  Frequencies=[]  NoiseDistribution=none  NoiseParameters=[]  Unit=1  AffineConversion=off  FilteringAndDerivatives=provide  SimscapeFilterOrder=1  InputFilterTimeConstant=0.001  UdotUserProvided=2
  Motion for PS : PMIOPort  Port=1  Side=Right
  wires:
  X/1 -> Simulink-PS Converter/1, Difference1/1
  Difference/1 -> Simulink-PS Converter/3
  Difference1/1 -> Difference/1, Simulink-PS Converter/2
  connections:
  Simulink-PS Converter/RConn1 -- Motion for PS/RConn1

== system AariaHIABTorqueR2017a2/Base/BaseVSS/BaseMotion/x 2motion7 ==
  X : Inport
  Difference : simulink/Discrete/Difference  ICPrevInput=1  InputProcessing=Inherited  OutMin=[]  OutMax=[]  OutDataType=fixdt(1, 16)  OutScaling=2^-10  DoSatur=off
  Difference1 : simulink/Discrete/Difference  ICPrevInput=0  InputProcessing=Inherited  OutMin=[]  OutMax=[]  OutDataType=fixdt(1, 16)  OutScaling=2^-10  DoSatur=off
  Simulink-PS Converter : nesl_utility/Simulink-PS Converter  PhysicalDomain=network_engine_domain  SubClassName=ps_input  LeftPortType=input  RightPortType=output  PseudoPeriodic=off  Frequencies=[]  NoiseDistribution=none  NoiseParameters=[]  Unit=1  AffineConversion=off  FilteringAndDerivatives=provide  SimscapeFilterOrder=1  InputFilterTimeConstant=0.001  UdotUserProvided=2
  Motion for PS : PMIOPort  Port=1  Side=Right
  wires:
  Difference1/1 -> Simulink-PS Converter/2, Difference/1
  Difference/1 -> Simulink-PS Converter/3
  X/1 -> Difference1/1, Simulink-PS Converter/1
  connections:
  Simulink-PS Converter/RConn1 -- Motion for PS/RConn1

== system AariaHIABTorqueR2017a2/Base/BaseVSS/BaseTorque/IMU Base ==
  Sensor Module1 : Subsystem  mask{nL=nL, nS=1}
      mask prompts: nL "Link Number"; nS "Sensor ID of that link"
      mask DialogControl DescGroupVar Prompt: Virtual IMU
      mask DialogControl DescTextVar Prompt: Measures Connected Body's acceleration and angular velocity in the given point
      mask DialogControl Control2 Prompt: The following numbers defines the corresponding numbers for this sensor to read from the parameters file
  Body Coord : PMIOPort  Port=1  Side=Left
  Reference Coord : PMIOPort  Port=2  Side=Left
  Out1 : Outport
  Out2 : Outport  Port=2
  Out3 : Outport  Port=3
  Out4 : Outport  Port=4
  wires:
  Sensor Module1/3(Out2) -> Out3/1
  Sensor Module1/2(Out4) -> Out2/1
  Sensor Module1/4(Out3) -> Out4/1
  Sensor Module1/1(Out5) -> Out1/1
  connections:
  Sensor Module1/LConn2 -- Reference Coord/RConn1
  Sensor Module1/LConn1 -- Body Coord/RConn1

== system AariaHIABTorqueR2017a2/Base/BaseVSS/BaseTorque/x 2motion2 ==
  X : Inport
  Difference : simulink/Discrete/Difference  ICPrevInput=1  InputProcessing=Inherited  OutMin=[]  OutMax=[]  OutDataType=fixdt(1, 16)  OutScaling=2^-10  DoSatur=off
  Difference1 : simulink/Discrete/Difference  ICPrevInput=0  InputProcessing=Inherited  OutMin=[]  OutMax=[]  OutDataType=fixdt(1, 16)  OutScaling=2^-10  DoSatur=off
  Simulink-PS Converter : nesl_utility/Simulink-PS Converter  PhysicalDomain=network_engine_domain  SubClassName=ps_input  LeftPortType=input  RightPortType=output  PseudoPeriodic=off  Frequencies=[]  NoiseDistribution=none  NoiseParameters=[]  Unit=1  AffineConversion=off  FilteringAndDerivatives=provide  SimscapeFilterOrder=1  InputFilterTimeConstant=0.001  UdotUserProvided=2
  Motion for PS : PMIOPort  Port=1  Side=Right
  wires:
  X/1 -> Simulink-PS Converter/1, Difference1/1
  Difference/1 -> Simulink-PS Converter/3
  Difference1/1 -> Difference/1, Simulink-PS Converter/2
  connections:
  Simulink-PS Converter/RConn1 -- Motion for PS/RConn1

== system AariaHIABTorqueR2017a2/Base/BaseVSS/BaseTorque/x 2motion3 ==
  X : Inport
  Difference : simulink/Discrete/Difference  ICPrevInput=1  InputProcessing=Inherited  OutMin=[]  OutMax=[]  OutDataType=fixdt(1, 16)  OutScaling=2^-10  DoSatur=off
  Difference1 : simulink/Discrete/Difference  ICPrevInput=0  InputProcessing=Inherited  OutMin=[]  OutMax=[]  OutDataType=fixdt(1, 16)  OutScaling=2^-10  DoSatur=off
  Simulink-PS Converter : nesl_utility/Simulink-PS Converter  PhysicalDomain=network_engine_domain  SubClassName=ps_input  LeftPortType=input  RightPortType=output  PseudoPeriodic=off  Frequencies=[]  NoiseDistribution=none  NoiseParameters=[]  Unit=1  AffineConversion=off  FilteringAndDerivatives=provide  SimscapeFilterOrder=1  InputFilterTimeConstant=0.001  UdotUserProvided=2
  Motion for PS : PMIOPort  Port=1  Side=Right
  wires:
  Difference1/1 -> Simulink-PS Converter/2, Difference/1
  Difference/1 -> Simulink-PS Converter/3
  X/1 -> Difference1/1, Simulink-PS Converter/1
  connections:
  Simulink-PS Converter/RConn1 -- Motion for PS/RConn1

== system AariaHIABTorqueR2017a2/Base/BaseVSS/BaseTorque/x 2motion4 ==
  X : Inport
  Difference : simulink/Discrete/Difference  ICPrevInput=1  InputProcessing=Inherited  OutMin=[]  OutMax=[]  OutDataType=fixdt(1, 16)  OutScaling=2^-10  DoSatur=off
  Difference1 : simulink/Discrete/Difference  ICPrevInput=0  InputProcessing=Inherited  OutMin=[]  OutMax=[]  OutDataType=fixdt(1, 16)  OutScaling=2^-10  DoSatur=off
  Simulink-PS Converter : nesl_utility/Simulink-PS Converter  PhysicalDomain=network_engine_domain  SubClassName=ps_input  LeftPortType=input  RightPortType=output  PseudoPeriodic=off  Frequencies=[]  NoiseDistribution=none  NoiseParameters=[]  Unit=1  AffineConversion=off  FilteringAndDerivatives=provide  SimscapeFilterOrder=1  InputFilterTimeConstant=0.001  UdotUserProvided=2
  Motion for PS : PMIOPort  Port=1  Side=Right
  wires:
  X/1 -> Simulink-PS Converter/1, Difference1/1
  Difference/1 -> Simulink-PS Converter/3
  Difference1/1 -> Difference/1, Simulink-PS Converter/2
  connections:
  Simulink-PS Converter/RConn1 -- Motion for PS/RConn1
